simulink model "modelos"  (R2016a)
settings: Solver=VariableStepAuto  StartTime=0.0  StopTime=10.0  MaxStep=0.01  RelTol=1e-3
values from neighbouring files (symbols this model uses):
  A = double(subs(jacobian(f),[x1 x2],[0 0]))    [Projeto.m]    (also in questao2.m = [0 1 0 0; questao3.m = double(subs(jacobian(f,x),[x1 x2 x3 x4],[0 0 0 0])))
  Am = M    (= 1)    [questao2.m]
  B = double(subs(u, [x1 x2],[0 0]))    [Projeto.m]    (also in questao2.m = [0; 1/M; 0; -1/(M*L)]; questao3.m = double(subs(uf,[x3 x4],[0 0])))
  Bm = N    [questao2.m]
  C = [1 0 0 ... (first row only)    [Projeto.m]    (also in questao2.m = [1 0 0 0]; questao3.m = [1 0 0 0])
  Dsim = zeros(4,1)    [questao2.m]
  K = place(A,B,P1)    [Projeto.m]    (also in questao2.m = Ka(:,1:4); questao3.m = place(A,B, [pd pd-.01 pd+0.05 pd+0.02]))
  Km = Ka(:,5:6)    [questao2.m]    (also in questao3.m = Kc(1,5))
  L = place(A',C',[pd pd-0.05 pd-0.03])'    [Projeto.m]    (also in pendulo_n_liear.m = 1; pendulo_n_linear.m = 1; questao2.m = H'; questao3.m = place(A',C',[pd pd-0.05 pd-0.03 pd-0.04])')
  x0 = [pi/180*180 0 0]    [Projeto.m]    (also in questao2.m = [0 0 pi/4 0]; questao3.m = [0 0 0.1 0])
  x0obs = [pi/4 ; 0; 0]    [Projeto.m]    (also in questao2.m = [0 0 0 0]; questao3.m = [0 ; 0; 0.1; 0])
settings Model: Creator=Regner  LastModifiedBy=Regner

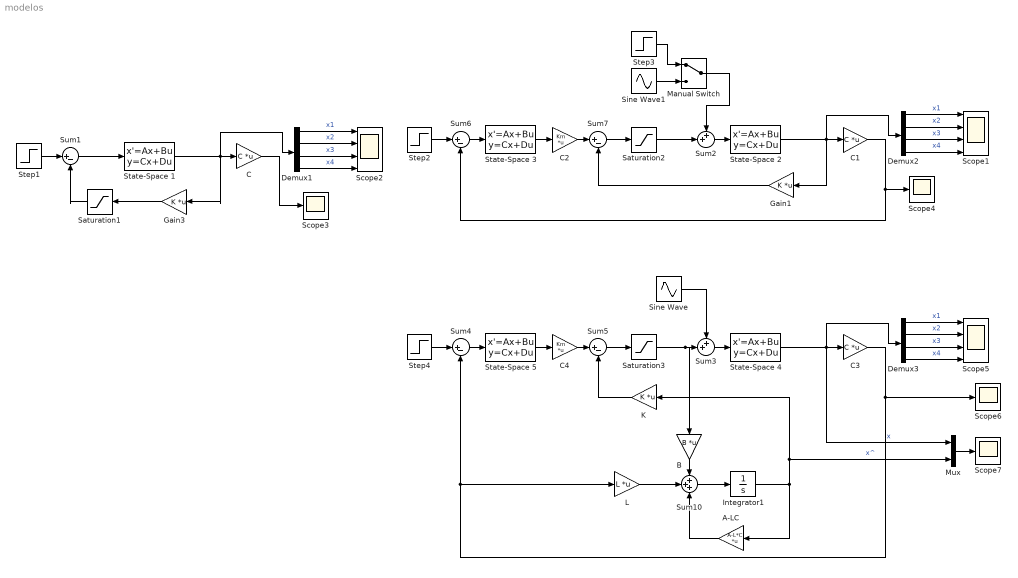
== system modelos ==
  A-LC : Gain  Gain=A-L*C  Multiplication=Matrix(K*u)
  B : Gain  Gain=B  Multiplication=Matrix(K*u)
  C : Gain  Gain=C  Multiplication=Matrix(K*u)
  C1 : Gain  Gain=C  Multiplication=Matrix(K*u)
  C2 : Gain  Gain=Km  Multiplication=Matrix(K*u)
  C3 : Gain  Gain=C  Multiplication=Matrix(K*u)
  C4 : Gain  Gain=Km  Multiplication=Matrix(K*u)
  Demux1 : Demux
  Demux2 : Demux
  Demux3 : Demux
  Gain1 : Gain  Gain=K  Multiplication=Matrix(K*u)
  Gain3 : Gain  Gain=K  Multiplication=Matrix(K*u)
  Integrator1 : Integrator  InitialCondition=x0obs
  K : Gain  Gain=K  Multiplication=Matrix(K*u)
  L : Gain  Gain=L  Multiplication=Matrix(K*u)
  Manual Switch : ManualSwitch
  Mux : Mux  Inputs=2
  Saturation1 : Saturate  UpperLimit=50  LowerLimit=-50
  Saturation2 : Saturate  UpperLimit=50  LowerLimit=-50
  Saturation3 : Saturate  UpperLimit=50  LowerLimit=-50
  Scope1 : Scope  NumInputPorts=4
  Scope2 : Scope  NumInputPorts=4
  Scope{3..4,6..7} (4 alike) : Scope
  Scope5 : Scope  NumInputPorts=4
  Sine Wave : Sin  Frequency=0.1  SampleTime=0
  Sine Wave1 : Sin  Frequency=0.1  SampleTime=0
  State-Space 1 : StateSpace  A=A  B=B  C=eye(4)  D=Dsim  X0=x0
  State-Space 2 : StateSpace  A=A  B=B  C=eye(4)  D=Dsim  X0=x0
  State-Space 3 : StateSpace  A=Am  B=Bm  C=eye(6)  D=zeros(6,2)  X0=0
  State-Space 4 : StateSpace  A=A  B=B  C=eye(4)  D=Dsim  X0=x0
  State-Space 5 : StateSpace  A=Am  B=Bm  C=eye(6)  D=zeros(6,2)  X0=0
  Step{1..4} (4 alike) : Step  Time=0  After=0  SampleTime=0
  Sum{1,4..7} (5 alike) : Sum  Inputs=|+-
  Sum10 : Sum  Inputs=+++
  Sum2 : Sum  Inputs=++|
  Sum3 : Sum  Inputs=++|
  wires:
  Demux1/1 -> Scope2/1  "x1"
  Demux1/2 -> Scope2/2  "x2"
  Demux1/3 -> Scope2/3  "x3"
  Demux1/4 -> Scope2/4  "x4"
  C/1 -> Scope3/1
  State-Space 1/1 -> C/1, Demux1/1, Gain3/1
  Step1/1 -> Sum1/1
  Sum1/1 -> State-Space 1/1
  Gain3/1 -> Saturation1/1
  Saturation1/1 -> Sum1/2
  Demux3/1 -> Scope5/1  "x1"
  Demux3/2 -> Scope5/2  "x2"
  Demux3/3 -> Scope5/3  "x3"
  Demux3/4 -> Scope5/4  "x4"
  State-Space 4/1 -> Mux/1, C3/1, Demux3/1  "x"
  Step4/1 -> Sum4/1
  Sum4/1 -> State-Space 5/1
  K/1 -> Sum5/2
  State-Space 5/1 -> C4/1
  C4/1 -> Sum5/1
  Sum3/1 -> State-Space 4/1
  Sine Wave/1 -> Sum3/1
  Sum5/1 -> Saturation3/1
  Demux2/1 -> Scope1/1  "x1"
  Demux2/2 -> Scope1/2  "x2"
  Demux2/3 -> Scope1/3  "x3"
  Demux2/4 -> Scope1/4  "x4"
  C1/1 -> Sum6/2, Scope4/1
  State-Space 2/1 -> Gain1/1, Demux2/1, C1/1
  Step2/1 -> Sum6/1
  Sum6/1 -> State-Space 3/1
  Gain1/1 -> Sum7/2
  State-Space 3/1 -> C2/1
  C2/1 -> Sum7/1
  Sum2/1 -> State-Space 2/1
  Manual Switch/1 -> Sum2/1
  Sum7/1 -> Saturation2/1
  Saturation2/1 -> Sum2/2
  Saturation3/1 -> B/1, Sum3/2
  C3/1 -> Sum4/2, L/1, Scope6/1
  Sum10/1 -> Integrator1/1
  L/1 -> Sum10/2
  A-LC/1 -> Sum10/3
  Integrator1/1 -> Mux/2, K/1, A-LC/1  "x^"
  B/1 -> Sum10/1
  Mux/1 -> Scope7/1
  Sine Wave1/1 -> Manual Switch/2
  Step3/1 -> Manual Switch/1
